simulink library "externalInputSensorProcessing"  (R2020a)
settings: Solver=VariableStepAuto  StartTime=0.0  StopTime=10.0  RelTol=1e-3
undefined symbols (not defined in the file or in its folder): flwSpd, initializeBussesFromBlock
settings Model: Creator=mcobb  LastModifiedBy=adabney
settings DataIOCC: ReturnWorkspaceOutputs=off
settings DebuggingCC: ArithmeticOperatorsInVariantConditions=warning
settings SFSimCC: CustomCodeUndefinedFunction=UseInterfaceOnly

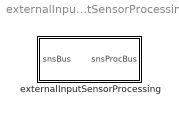
== system externalInputSensorProcessing ==
  externalInputSensorProcessing : Subsystem  LoadFcn=initializeBussesFromBlock(gcb)  InitFcn=initializeBussesFromBlock(gcb)  StartFcn=initializeBussesFromBlock(gcb)

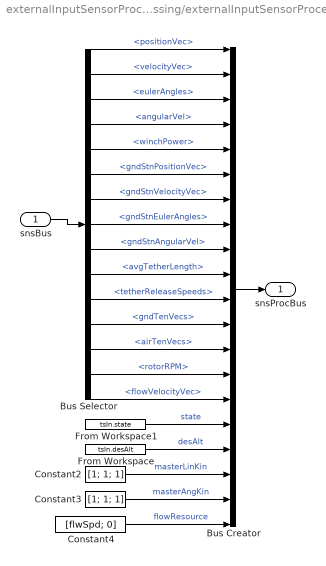
== system externalInputSensorProcessing/externalInputSensorProcessing ==
  snsBus : Inport  OutDataTypeStr=Bus: sensorsBus
  Bus Creator : BusCreator  Inputs=20  OutDataTypeStr=Bus: sensorsProcessingBus  NonVirtualBus=on
  Bus Selector : BusSelector  OutputSignals=positionVec,velocityVec,eulerAngles,angularVel,winchPower,gndStnPositionVec,gndStnVelocityVec,gndStnEulerAngles,gndStnAngularVel,avgTetherLength,tetherReleaseSpeeds,gndTenVecs,airTenVecs,rotorRPM,flowVelocityVec
  Constant2 : Constant  Value=[1; 1; 1]
  Constant3 : Constant  Value=[1; 1; 1]
  Constant4 : Constant  Value=[flwSpd; 0]
  From Workspace : FromWorkspace  VariableName=tsIn.desAlt
  From Workspace1 : FromWorkspace  VariableName=tsIn.state
  snsProcBus : Outport  OutDataTypeStr=Bus: sensorsProcessingBus  VectorParamsAs1DForOutWhenUnconnected=off
  wires:
  snsBus/1 -> Bus Selector/1
  Bus Creator/1 -> snsProcBus/1
  Bus Selector/1 -> Bus Creator/1  "<positionVec>"
  Bus Selector/2 -> Bus Creator/2  "<velocityVec>"
  Bus Selector/3 -> Bus Creator/3  "<eulerAngles>"
  Bus Selector/4 -> Bus Creator/4  "<angularVel>"
  Bus Selector/5 -> Bus Creator/5  "<winchPower>"
  Bus Selector/6 -> Bus Creator/6  "<gndStnPositionVec>"
  Bus Selector/7 -> Bus Creator/7  "<gndStnVelocityVec>"
  Bus Selector/8 -> Bus Creator/8  "<gndStnEulerAngles>"
  Bus Selector/9 -> Bus Creator/9  "<gndStnAngularVel>"
  Bus Selector/10 -> Bus Creator/10  "<avgTetherLength>"
  Bus Selector/11 -> Bus Creator/11  "<tetherReleaseSpeeds>"
  Bus Selector/12 -> Bus Creator/12  "<gndTenVecs>"
  Bus Selector/15 -> Bus Creator/15  "<flowVelocityVec>"
  Bus Selector/13 -> Bus Creator/13  "<airTenVecs>"
  Bus Selector/14 -> Bus Creator/14  "<rotorRPM>"
  From Workspace1/1 -> Bus Creator/16  "state"
  From Workspace/1 -> Bus Creator/17  "desAlt"
  Constant2/1 -> Bus Creator/18  "masterLinKin"
  Constant3/1 -> Bus Creator/19  "masterAngKin"
  Constant4/1 -> Bus Creator/20  "flowResource"
